simulink model "IM_VF_Control"  (R2014a)
settings: Solver=ode23tb  StartTime=0  StopTime=1  MaxStep=50e-6  RelTol=1e-3
libraries: powerlib x5, powerlib_meascontrol x1
settings Model: Creator=Admin  LastModifiedBy=ninad gaikawad
settings DebuggingCC: UnderspecifiedInitializationDetection=Classic  StateNameClashWarn=warning

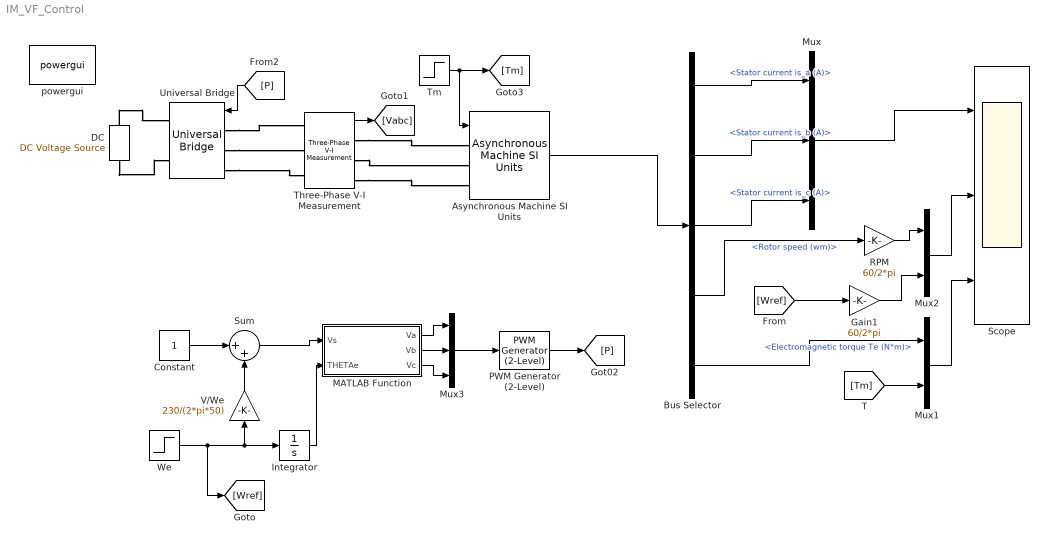
== system IM_VF_Control ==
  Asynchronous Machine SI Units : powerlib/Machines/Asynchronous Machine SI Units  PresetModel="15:  5.4 HP (4KW)   400 V  50Hz 1430 RPM"  MechanicalLoad=Torque Tm  ShowDetailedParameters=on  RotorType=Squirrel-cage  ReferenceFrame=Rotor  Units=SI  MeasurementBus=off  NominalParameters=[4000 400 50]  Stator=[1.405 0.005839]  Rotor=[1.395 0.005839]  Cage1=[ 0.022 0.226/377]  Cage2=[ 0.022 0.226/377]  Lm=0.1722  Mechanical=[0.0131 0.002985 2]  PolePairs=2  InitialConditions=[1 0 0 0 0 0 0 0]  SimulateSaturation=off  Saturation=[14.03593122, 27.81365428, 53.79336849, 72.68890987, 97.98006896, 148.6815601, 215.7428561, 302.9841135, 420.4778367 ; 230, 322, 414, 460, 506, 552, 598, 644, 690]  LoadFlowParameters=1492000  TsPowergui=0  TsBlock=-1  IterativeModel=Trapezoidal non iterative  Pmec=0
  Bus Selector : BusSelector  OutputSignals=Stator measurements.Stator current is_a (A),Stator measurements.Stator current is_b (A),Stator measurements.Stator current is_c (A),Mechanical.Rotor speed (wm),Mechanical.Electromagnetic torque Te (N*m)
  Constant : Constant
  "DC " : powerlib/Electrical Sources/DC Voltage Source  Amplitude=565.7  Measurements=None
  Gain1 : Gain  Gain=60/2*pi
  Integrator : Integrator
  MATLAB Function : MATLAB Function  TreatAsAtomicUnit=on
  Mux : Mux  Inputs=3
  Mux1 : Mux  Inputs=2
  Mux2 : Mux  Inputs=2
  Mux3 : Mux  Inputs=3
  PWM Generator (2-Level) : powerlib_meascontrol/Pulse & Signal Generators/PWM Generator (2-Level)  ModulatorType=Three-phase bridge (6 pulses)  ModulatorMode=Unsynchronized  nF=27  Fc=4000  ModulatingSignals=off  m=0.8  Freq=60  Phase=0  Ts=0
  RPM : Gain  Gain=60/2*pi
  Scope : Scope  NumInputPorts=3
      settings: YMin=-5~-5~-5  YMax=5~5~5
  Sum : Sum  Inputs=|++
  Three-Phase V-I Measurement : powerlib/Measurements/Three-Phase V-I Measurement  VoltageMeasurement=phase-to-phase  SetLabelV=off  LabelV=Vabc  Vpu=off  VpuLL=off  CurrentMeasurement=no  SetLabelI=off  LabelI=Iabc  Ipu=off  Pbase=100e6  Vbase=500e3  OutputType=Complex  PhasorSimulation=off  PSBequivalent=0
  Tm : Step  Time=0.3  Before=26.71*0.5  After=26.71  SampleTime=0
  Universal Bridge : powerlib/Power Electronics/Universal Bridge  Arms=3  SnubberResistance=1e5  SnubberCapacitance=inf  Device=IGBT / Diodes  Ron=1e-6  Lon=0  ForwardVoltages="[  0  0  ]"  ForwardVoltage=0  GTOparameters=[ 10e-6 , 20e-6 ]  IGBTparameters=[ 1e-6 , 2e-6 ]  Measurements=None  Measurements_2=None  converterType=Rectifier
  V/We : Gain  Gain=230/(2*pi*50)
  We : Step  Time=0.5  Before=2*pi*50  After=2*pi*50*0.5  SampleTime=0
  powergui : powerlib/powergui  Priority=1  SimulationMode=Continuous  SolverType=Tustin  SampleTime=50e-6  frequency=60  SPID=off  DisableSnubberDevices=off  DisableRonSwitches=off  DisableVfSwitches=off  SwTol=0  Interpol=off  DisplayEquations=off  Ts=0  methode=off  frequencyindice=50  Pbase=100e6  ErrMax=1e-4  Iterations=50  UnitsV=kV  UnitsW=MW  FunctionMessages=off  echomessages=off  HookPort=off  EnableUseOfTLC=off  x0status=blocks  RestoreLinks=warning  ResistiveCurrentMeasurement=off  Frange=[0:2:500]  Ylog=off  Xlog=on  ShowGrid=off  save=off  variable=ZData  structure=0  ZoomFFT=off  StartTime=0.0  cycles=1  DisplayStyle=1  fundamental=60  FreqAxis=off  MaxFrequency=1000  frequencyindicesteady=1  RmsSteady=1  display=off
  wires:
  Asynchronous Machine SI Units/1 -> Bus Selector/1
  [Wref] -> Gain1/1
  RPM/1 -> Mux2/1
  [Tm] -> Mux1/2
  Mux1/1 -> Scope/3
  Mux2/1 -> Scope/2
  [P] -> Universal Bridge/1
  Constant/1 -> Sum/1
  V/We/1 -> Sum/2
  Sum/1 -> MATLAB Function/1(Vs)
  MATLAB Function/3(Vc) -> Mux3/3
  MATLAB Function/2(Vb) -> Mux3/2
  MATLAB Function/1(Va) -> Mux3/1
  Mux3/1 -> PWM Generator (2-Level)/1
  PWM Generator (2-Level)/1 -> [P]
  We/1 -> [Wref], V/We/1, Integrator/1
  Integrator/1 -> MATLAB Function/2(THETAe)
  Three-Phase V-I Measurement/1 -> [Vabc]
  Tm/1 -> Asynchronous Machine SI Units/1, [Tm]
  Bus Selector/1 -> Mux/1  "<Stator current is_a (A)>"
  Bus Selector/2 -> Mux/2  "<Stator current is_b (A)>"
  Bus Selector/3 -> Mux/3  "<Stator current is_c (A)>"
  Bus Selector/4 -> RPM/1  "<Rotor speed (wm)>"
  Bus Selector/5 -> Mux1/1  "<Electromagnetic torque Te (N*m)>"
  Mux/1 -> Scope/1
  Gain1/1 -> Mux2/2
  connections:
  "DC "/RConn1 -- Universal Bridge/RConn1
  "DC "/LConn1 -- Universal Bridge/RConn2
  Universal Bridge/LConn2 -- Three-Phase V-I Measurement/LConn2
  Universal Bridge/LConn3 -- Three-Phase V-I Measurement/LConn3
  Three-Phase V-I Measurement/RConn1 -- Asynchronous Machine SI Units/LConn1
  Three-Phase V-I Measurement/RConn2 -- Asynchronous Machine SI Units/LConn2
  Three-Phase V-I Measurement/RConn3 -- Asynchronous Machine SI Units/LConn3
  Universal Bridge/LConn1 -- Three-Phase V-I Measurement/LConn1

== matlab function IM_VF_Control/MATLAB Function ==
  data: Vs input; Va output; THETAe input; Vb output; Vc output
function [Va,Vb,Vc] = fcn(Vs,THETAe)
 Va=[sqrt(2)*Vs*sin(THETAe)]/326;
 Vb=[sqrt(2)*Vs*sin(THETAe-(2*pi/3))]/326;
 Vc=[sqrt(2)*Vs*sin(THETAe+(2*pi/3))]/326; 
 
%#codegen
